simulink model "Vi"  (R2022b)
settings: Solver=FixedStepAuto  StartTime=0.0  StopTime=10.0  RelTol=1e-3
settings Model: Creator=86134  LastModifiedBy=86134

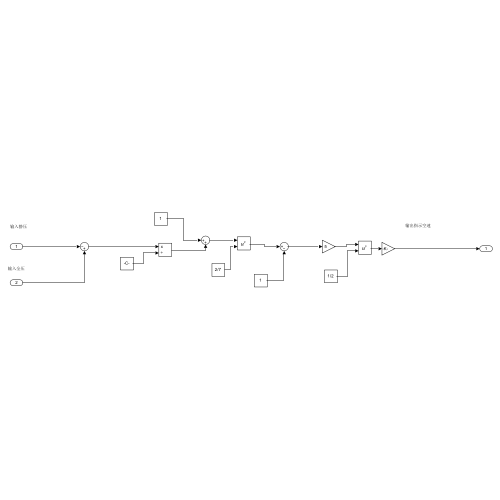
[thumbnail: Simulink's stored preview of the top-level diagram]
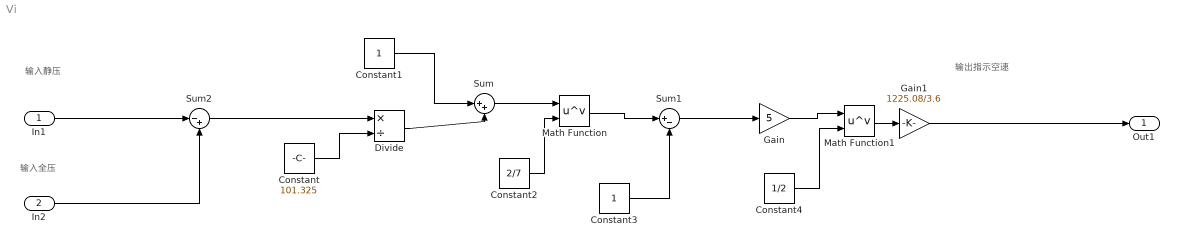
== system Vi ==
  note: 输入静压
  note: 输入全压
  note: 输出指示空速
  In1 : Inport
  In2 : Inport  Port=2
  Constant : Constant  Value=101.325
  Constant1 : Constant
  Constant2 : Constant  Value=2/7
  Constant3 : Constant
  Constant4 : Constant  Value=1/2
  Divide : Product  Inputs=*/
  Gain : Gain  Gain=5
  Gain1 : Gain  Gain=1225.08/3.6
  Math Function : Math  Operator=pow
  Math Function1 : Math  Operator=pow
  Sum : Sum  Inputs=|++
  Sum1 : Sum  Inputs=|+-
  Sum2 : Sum  Inputs=|-+
  Out1 : Outport
  wires:
  Constant/1 -> Divide/2
  Sum2/1 -> Divide/1
  Constant1/1 -> Sum/1
  Divide/1 -> Sum/2
  Sum/1 -> Math Function/1
  Constant2/1 -> Math Function/2
  Math Function/1 -> Sum1/1
  Constant3/1 -> Sum1/2
  Sum1/1 -> Gain/1
  Gain/1 -> Math Function1/1
  Constant4/1 -> Math Function1/2
  Math Function1/1 -> Gain1/1
  Gain1/1 -> Out1/1
  In2/1 -> Sum2/2
  In1/1 -> Sum2/1
